simulink model "Dvig2016"  (R2021b)
settings: Solver=VariableStepAuto  StartTime=0.0  StopTime=20  RelTol=1e-3
values from neighbouring files (symbols this model uses):
  ke = U/w    (= 0.690310596543)    [Init.m]
  km = i*(M/I)    (= 24.1911764706)    [Init.m]
  Tm = (J*w)/M0    (= 0.000140723404261)    [Init.m]
settings Model: Creator=Адель  LastModifiedBy=Адель
settings DebuggingCC: UnconnectedInputMsg=none  UnconnectedOutputMsg=none  UnconnectedLineMsg=none
settings RTWCC: DLArmComputeVersion=20.02.1

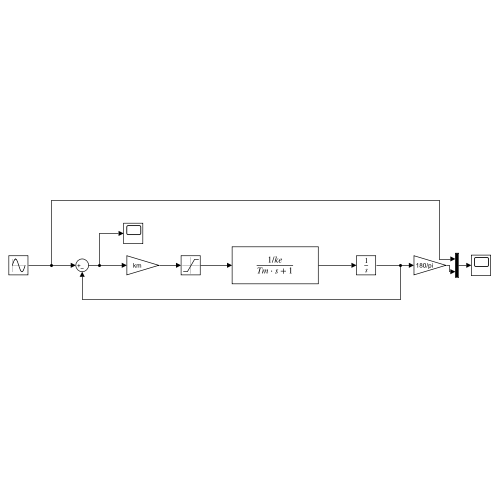
[thumbnail: Simulink's stored preview of the top-level diagram]
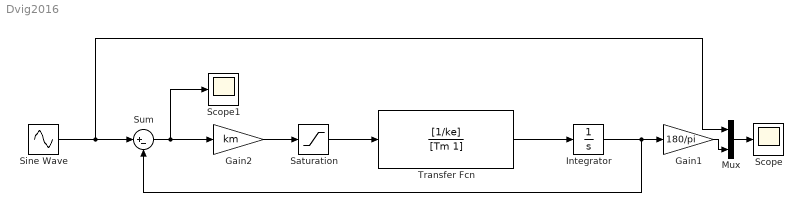
== system Dvig2016 ==
  Gain1 : Gain  Gain=180/pi
  Gain2 : Gain  Gain=km
  Integrator : Integrator
  Mux : Mux  Inputs=2
  Saturation : Saturate  UpperLimit=2  LowerLimit=-2  LinearizeAsGain=off
  Scope : Scope
  Scope1 : Scope
  Sine Wave : Sin  SampleTime=0
  Sum : Sum  Inputs=|+-
  Transfer Fcn : TransferFcn  Numerator=[1/ke]  Denominator=[Tm 1]
  wires:
  Sine Wave/1 -> Mux/1, Sum/1
  Sum/1 -> Gain2/1, Scope1/1
  Transfer Fcn/1 -> Integrator/1
  Integrator/1 -> Sum/2, Gain1/1
  Saturation/1 -> Transfer Fcn/1
  Gain2/1 -> Saturation/1
  Gain1/1 -> Mux/2
  Mux/1 -> Scope/1
